simulink model "gm_sampleModel1847_5_sub"  (R2023a)
settings: Solver=VariableStepAuto  StartTime=0.0  StopTime=10.0  RelTol=1e-3
libraries: hdlsllib x1
settings Model: Creator=user1  LastModifiedBy=user1
settings OptimizationCC: BlockReduction=off  ConditionallyExecuteInputs=off
settings DebuggingCC: InheritedTsInSrcMsg=none

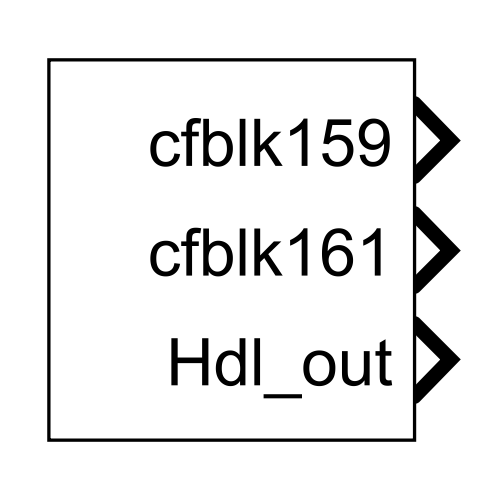
[thumbnail: Simulink's stored preview of the top-level diagram]
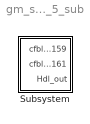
== system gm_sampleModel1847_5_sub ==
  Subsystem : Subsystem

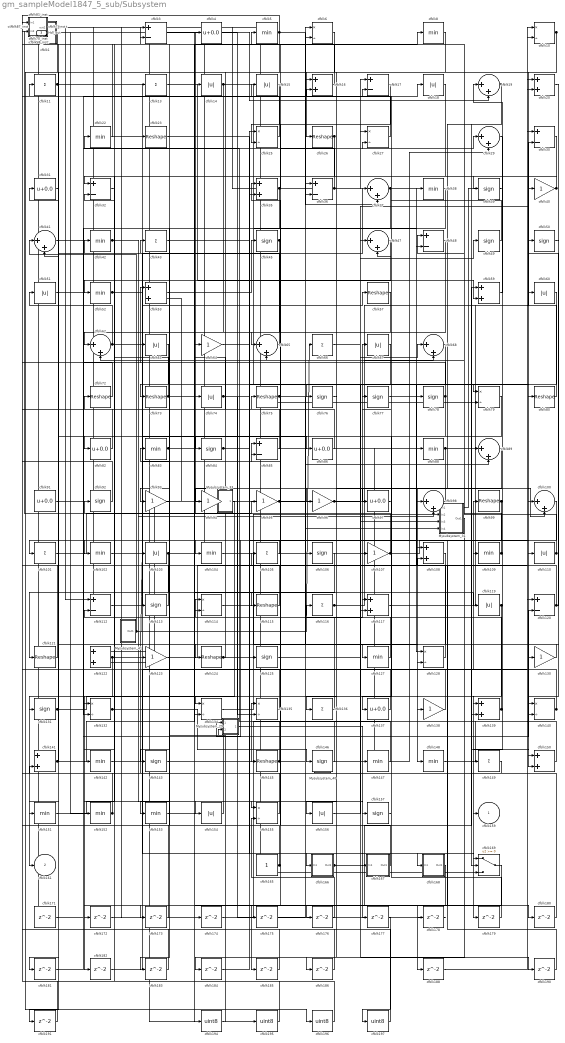
== system gm_sampleModel1847_5_sub/Subsystem ==
  Mysubsystem_29 : Subsystem
  Mysubsystem_31 : Subsystem
  Mysubsystem_33 : Subsystem
  Mysubsystem_40 : Subsystem
  Mysubsystem_41 : Subsystem
  cfblk1 : Subsystem  mask(Detect Fall Nonpositive){vinit=double(0), InputProcessing=Elements as channels (sample based), OutDataTypeStr=uint8}
      mask prompts: vinit "Simulink:masks:InitialCondition_MP"; InputProcessing "Simulink:masks:InputProcessing_MP"; OutDataTypeStr "Simulink:masks:OutputDataType_MP"
      mask help: Simulink:masks:DetectFallNonpositive_MD
      mask init:
      | InputProcessing = 'Elements as channels (sample based)';
      | OutDataTypeStr = 'uint8';
      | vinit = double(0);
      mask TypeOptions InputProcessing: Simulink:masks:ColumnsAsChannelsFrameBased | Simulink:masks:ElementsAsChannelsSampleBased
      mask TypeOptions OutDataTypeStr: Simulink:masks:uint8 | Simulink:masks:boolean
      mask Display: fprintf('U <= 0\n&  NOT\nU/z <= 0')
  cfblk{6,10,25,27,79,114,128,132,134..135,140,155} (12 alike) : Product  Inputs=*/  OutDataTypeStr=uint8  RndMeth=Zero  SaturateOnIntegerOverflow=on
  cfblk{19,29,37,41,47,62,65,68,89,98,100} (11 alike) : Sum  Inputs=|++  OutDataTypeStr=uint8
  cfblk{11,13,43,66,101,105,116,136,149} (9 alike) : Sum  Inputs=+  OutDataTypeStr=uint8
  cfblk{5,8,22,38,42,52,83,88,102,104,109,127,142,147..148,151..153} (18 alike) : MinMax  OutDataTypeStr=uint8
  cfblk{14..15,18,51,60,63,67,74,103,110,119,154,156} (13 alike) : Abs  OutDataTypeStr=uint8  SaturateOnIntegerOverflow=off
  cfblk{39,45,49..50,76..78,84,92,106,113,125,131,143,146,157} (16 alike) : Signum
  cfblk{40,64,93..96,107,123,130,138} (10 alike) : Gain  OutDataTypeStr=uint8
  cfblk{16,20,35,53,59,108,117,122,139,141,150} (11 alike) : Sum  OutDataTypeStr=uint8
  cfblk{3,17,30,32,36,48,85,112,120} (9 alike) : Sum  Inputs=+-  OutDataTypeStr=uint8
  cfblk{23,26,57,72..73,75,80,99,115,121,124,145} (12 alike) : Reshape
  cfblk12_inst : Subsystem
  cfblk133_inst : Subsystem
  cfblk{4,31,82,86,91,97,137} (7 alike) : Bias  Bias=0.0  SaturateOnIntegerOverflow=off
  cfblk144_inst : Subsystem
  cfblk165 : Constant  OutDataTypeStr=uint8  SampleTime=-1
  cfblk166 : Subsystem
  cfblk167 : Subsystem
  cfblk168 : Subsystem
  cfblk169 : Switch  OutDataTypeStr=uint8  SaturateOnIntegerOverflow=off  InputSameDT=off
  cfblk{171..186,188,190..191} (19 alike) : Delay  SampleTime=1
  cfblk{194..197} (4 alike) : DataTypeConversion  OutDataTypeStr=uint8  SaturateOnIntegerOverflow=off  RndMeth=Floor
  cfblk24_inst : Subsystem
  cfblk34_inst : Subsystem
  cfblk55_inst : Subsystem
  cfblk56_inst : Subsystem
  cfblk58_inst : Subsystem
  cfblk70_inst : Subsystem
  cfblk7_inst : Subsystem
  cfblk81_inst : Subsystem
  cfblk87_inst : Subsystem
  cfblk159 : Outport  OutDataTypeStr=uint8  SampleTime=1  VectorParamsAs1DForOutWhenUnconnected=off
  cfblk161 : Outport  Port=2  OutDataTypeStr=uint8  SampleTime=1  VectorParamsAs1DForOutWhenUnconnected=off
  Hdl_out : Outport  Port=3  OutDataTypeStr=uint8  SampleTime=1
  wires:
  Mysubsystem_29/1(Out1) -> cfblk177/1
  Mysubsystem_31/1(Out1) -> cfblk184/1
  Mysubsystem_33/1(cfblk161) -> cfblk161/1
  Mysubsystem_40/1(Out1) -> cfblk29/2, cfblk88/1
  Mysubsystem_41/1(Out1) -> cfblk41/1, cfblk66/1
  cfblk1/1(Y) -> cfblk196/1
  cfblk10/1 -> cfblk26/1, cfblk150/2
  cfblk100/1 -> cfblk104/1
  cfblk101/1 -> cfblk95/1
  cfblk102/1 -> cfblk85/1
  cfblk103/1 -> cfblk181/1, cfblk180/1
  cfblk104/1 -> cfblk127/1
  cfblk105/1 -> cfblk101/1
  cfblk106/1 -> cfblk121/1
  cfblk107/1 -> cfblk81_inst/2(in2), cfblk4/1, cfblk110/1
  cfblk108/1 -> cfblk151/1
  cfblk109/1 -> cfblk55_inst/2(in2), cfblk48/1
  cfblk11/1 -> cfblk86/1, cfblk16/2, cfblk157/1
  cfblk110/1 -> cfblk87_inst/2(in2), cfblk62/2
  cfblk112/1 -> cfblk57/1
  cfblk113/1 -> cfblk56_inst/1(in1)
  cfblk114/1 -> Mysubsystem_31/2(In2)
  cfblk115/1 -> cfblk105/1
  cfblk116/1 -> cfblk68/2, cfblk30/2
  cfblk117/1 -> cfblk60/1
  cfblk119/1 -> cfblk179/1, cfblk159/1
  cfblk12_inst/1(out1) -> cfblk13/1
  cfblk120/1 -> cfblk75/1, cfblk50/1
  cfblk121/1 -> cfblk87_inst/1(in1)
  cfblk122/1 -> cfblk103/1, cfblk182/1
  cfblk123/1 -> cfblk20/1
  cfblk124/1 -> cfblk78/1, cfblk74/1
  cfblk125/1 -> Mysubsystem_31/3(In3)
  cfblk127/1 -> cfblk116/1
  cfblk128/1 -> cfblk3/1
  cfblk13/1 -> cfblk59/2
  cfblk130/1 -> cfblk124/1
  cfblk131/1 -> cfblk139/1, cfblk134/1
  cfblk132/1 -> cfblk194/1, cfblk146/1
  cfblk133_inst/1(out1) -> cfblk174/1
  cfblk134/1 -> cfblk99/1
  cfblk135/1 -> cfblk51/1
  cfblk136/1 -> cfblk112/2
  cfblk137/1 -> cfblk144_inst/1(in1)
  cfblk138/1 -> cfblk92/1
  cfblk139/1 -> cfblk67/1, cfblk47/2
  cfblk14/1 -> cfblk48/2, cfblk132/1, cfblk147/1
  cfblk140/1 -> cfblk85/2, cfblk109/1
  cfblk141/1 -> cfblk31/1, cfblk8/1
  cfblk142/1 -> cfblk169/1
  cfblk143/1 -> cfblk135/1
  cfblk144_inst/1(out1) -> cfblk12_inst/2(in2), cfblk38/1
  cfblk145/1 -> cfblk89/2, cfblk72/1, cfblk65/2, cfblk117/1, Mysubsystem_31/4(In4)
  cfblk146/1 -> cfblk22/1
  cfblk147/1 -> cfblk114/1
  cfblk148/1 -> cfblk120/2
  cfblk149/1 -> cfblk141/2
  cfblk15/1 -> cfblk25/2
  cfblk150/1 -> cfblk30/1
  cfblk151/1 -> cfblk154/1
  cfblk152/1 -> cfblk133_inst/2(in2), Hdl_out/1
  cfblk153/1 -> cfblk168/1(In1)
  cfblk154/1 -> cfblk83/1
  cfblk155/1 -> cfblk123/1
  cfblk156/1 -> cfblk49/1
  cfblk157/1 -> cfblk77/1
  cfblk16/1 -> cfblk7_inst/2(in2)
  cfblk165/1 -> cfblk32/2, cfblk43/1
  cfblk166/1(Out1) -> cfblk139/2, cfblk188/1
  cfblk167/1(Out1) -> cfblk35/1
  cfblk168/1(Out1) -> cfblk172/1
  cfblk169/1 -> cfblk185/1
  cfblk17/1 -> cfblk65/1
  cfblk171/1 -> cfblk140/2
  cfblk172/1 -> cfblk36/1
  cfblk173/1 -> cfblk34_inst/1(in1)
  cfblk174/1 -> cfblk20/2
  cfblk175/1 -> cfblk6/2
  cfblk176/1 -> cfblk155/2
  cfblk177/1 -> cfblk197/1
  cfblk178/1 -> cfblk1/1(U)
  cfblk179/1 -> cfblk17/2
  cfblk18/1 -> cfblk76/1
  cfblk180/1 -> cfblk59/1
  cfblk181/1 -> cfblk27/2
  cfblk182/1 -> cfblk10/2
  cfblk183/1 -> cfblk81_inst/1(in1)
  cfblk184/1 -> cfblk35/2
  cfblk185/1 -> cfblk12_inst/1(in1)
  cfblk186/1 -> cfblk144_inst/2(in2)
  cfblk188/1 -> cfblk120/1
  cfblk19/1 -> cfblk169/2, cfblk148/1
  cfblk190/1 -> cfblk108/2
  cfblk191/1 -> cfblk56_inst/2(in2)
  cfblk194/1 -> Mysubsystem_29/2(In2)
  cfblk195/1 -> cfblk42/1
  cfblk196/1 -> cfblk58_inst/1(in1)
  cfblk197/1 -> cfblk58_inst/2(in2)
  cfblk20/1 -> cfblk140/1
  cfblk22/1 -> cfblk7_inst/1(in1)
  cfblk23/1 -> cfblk97/1
  cfblk24_inst/1(out1) -> cfblk89/1, cfblk112/1
  cfblk25/1 -> cfblk24_inst/2(in2)
  cfblk26/1 -> cfblk62/1, cfblk36/2
  cfblk27/1 -> cfblk6/1
  cfblk29/1 -> cfblk149/1
  cfblk3/1 -> cfblk166/1(In1)
  cfblk30/1 -> cfblk152/1
  cfblk31/1 -> cfblk131/1
  cfblk32/1 -> cfblk142/1
  cfblk34_inst/1(out1) -> cfblk113/1
  cfblk35/1 -> cfblk82/1, cfblk132/2, cfblk5/1
  cfblk36/1 -> cfblk17/1, cfblk15/1
  cfblk37/1 -> cfblk100/2, cfblk93/1
  cfblk38/1 -> cfblk153/1
  cfblk39/1 -> Mysubsystem_31/1(In1)
  cfblk4/1 -> cfblk19/2
  cfblk40/1 -> cfblk39/1, cfblk32/1
  cfblk41/1 -> cfblk29/1
  cfblk42/1 -> cfblk98/2, cfblk155/1
  cfblk43/1 -> cfblk145/1
  cfblk45/1 -> cfblk183/1, cfblk52/1
  cfblk47/1 -> cfblk134/2
  cfblk48/1 -> cfblk102/1
  cfblk49/1 -> cfblk14/1
  cfblk5/1 -> cfblk55_inst/1(in1), cfblk41/2, cfblk37/2
  cfblk50/1 -> cfblk130/1
  cfblk51/1 -> cfblk18/1
  cfblk52/1 -> cfblk106/1, cfblk114/2
  cfblk53/1 -> cfblk45/1
  cfblk55_inst/1(out1) -> cfblk23/1
  cfblk56_inst/1(out1) -> cfblk107/1
  cfblk57/1 -> cfblk175/1
  cfblk58_inst/1(out1) -> cfblk195/1
  cfblk59/1 -> cfblk19/1
  cfblk6/1 -> cfblk84/1
  cfblk60/1 -> cfblk94/1
  cfblk62/1 -> cfblk37/1, cfblk11/1
  cfblk63/1 -> cfblk73/1
  cfblk64/1 -> cfblk80/1
  cfblk65/1 -> cfblk34_inst/2(in2)
  cfblk66/1 -> cfblk47/1
  cfblk67/1 -> cfblk115/1
  cfblk68/1 -> cfblk143/1
  cfblk7_inst/1(out1) -> cfblk91/1
  cfblk70_inst/1(out1) -> cfblk125/1
  cfblk72/1 -> cfblk70_inst/1(in1)
  cfblk73/1 -> cfblk133_inst/1(in1), cfblk117/2
  cfblk74/1 -> cfblk108/1, cfblk135/2
  cfblk75/1 -> cfblk16/1, cfblk128/2
  cfblk76/1 -> cfblk136/1
  cfblk77/1 -> cfblk79/1
  cfblk78/1 -> cfblk53/1, cfblk191/1, cfblk128/1
  cfblk79/1 -> cfblk137/1
  cfblk8/1 -> cfblk176/1
  cfblk80/1 -> cfblk10/1
  cfblk81_inst/1(out1) -> cfblk79/2, cfblk171/1
  cfblk82/1 -> cfblk24_inst/1(in1)
  cfblk83/1 -> cfblk3/2, cfblk96/1, cfblk27/1
  cfblk84/1 -> cfblk138/1, cfblk167/1(In1)
  cfblk85/1 -> cfblk64/1
  cfblk86/1 -> cfblk25/1
  cfblk87_inst/1(out1) -> cfblk169/3, cfblk141/1
  cfblk88/1 -> cfblk156/1, cfblk150/1
  cfblk89/1 -> cfblk98/1
  cfblk91/1 -> cfblk63/1
  cfblk92/1 -> cfblk70_inst/2(in2)
  cfblk93/1 -> cfblk173/1
  cfblk94/1 -> cfblk53/2, cfblk122/2, cfblk122/1
  cfblk95/1 -> cfblk119/1, cfblk100/1
  cfblk96/1 -> cfblk68/1, cfblk40/1, cfblk190/1
  cfblk97/1 -> Mysubsystem_33/1(u)
  cfblk98/1 -> cfblk186/1
  cfblk99/1 -> cfblk178/1, Mysubsystem_29/1(In1)

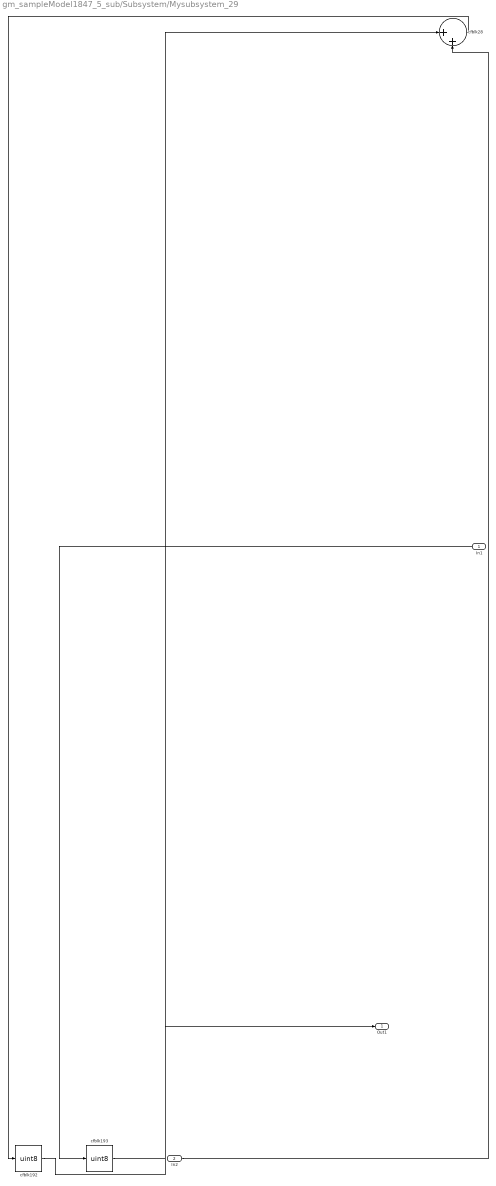
== system gm_sampleModel1847_5_sub/Subsystem/Mysubsystem_29 ==
  In1 : Inport  OutDataTypeStr=uint8  PortDimensions=1  SampleTime=1
  In2 : Inport  Port=2  OutDataTypeStr=uint8  PortDimensions=1  SampleTime=1
  cfblk192 : DataTypeConversion  OutDataTypeStr=uint8  SaturateOnIntegerOverflow=off  RndMeth=Floor
  cfblk193 : DataTypeConversion  OutDataTypeStr=uint8  SaturateOnIntegerOverflow=off  RndMeth=Floor
  cfblk28 : Sum  Inputs=|++
  Out1 : Outport  SampleTime=1
  wires:
  In1/1 -> cfblk193/1
  In2/1 -> cfblk28/2
  cfblk192/1 -> Out1/1
  cfblk193/1 -> cfblk28/1
  cfblk28/1 -> cfblk192/1

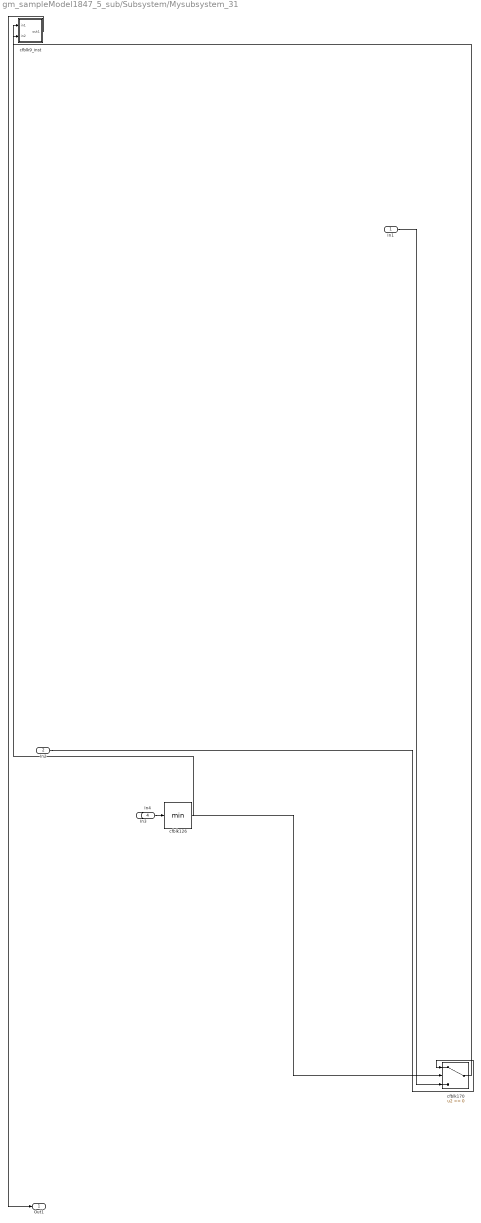
== system gm_sampleModel1847_5_sub/Subsystem/Mysubsystem_31 ==
  In1 : Inport  OutDataTypeStr=uint8  PortDimensions=1  SampleTime=1
  In2 : Inport  Port=2  OutDataTypeStr=uint8  PortDimensions=1  SampleTime=1
  In3 : Inport  Port=3  OutDataTypeStr=uint8  PortDimensions=1  SampleTime=1
  In4 : Inport  Port=4  OutDataTypeStr=uint8  PortDimensions=1  SampleTime=1
  cfblk126 : MinMax
  cfblk170 : Switch  SaturateOnIntegerOverflow=off  InputSameDT=off
  cfblk9_inst : Subsystem
  Out1 : Outport  SampleTime=1
  wires:
  In1/1 -> cfblk170/3
  In2/1 -> cfblk170/1
  In3/1 -> cfblk170/2
  In4/1 -> cfblk126/1
  cfblk126/1 -> cfblk9_inst/1(in1)
  cfblk170/1 -> cfblk9_inst/2(in2)
  cfblk9_inst/1(out1) -> Out1/1

== system gm_sampleModel1847_5_sub/Subsystem/Mysubsystem_33 ==
  u : Inport  OutDataTypeStr=uint8  PortDimensions=1  SampleTime=1
  cfblk2 : hdlsllib/Logic and Bit Operations/Bit Slice  lidx=7  ridx=0
  cfblk161 : Outport  SampleTime=1  VectorParamsAs1DForOutWhenUnconnected=off
  wires:
  u/1 -> cfblk2/1
  cfblk2/1 -> cfblk161/1

== system gm_sampleModel1847_5_sub/Subsystem/Mysubsystem_40 ==
  cfblk129 : Abs  SaturateOnIntegerOverflow=off
  cfblk163 : Subsystem  mask(Counter Limited){uplimit=double(7), tsamp=double(-1)}
      mask prompts: uplimit "Simulink:masks:UpperLimit_MP"; tsamp "Simulink:masks:SampleTime_MP"
      mask help: Simulink:masks:CounterLimited_MD
      mask init:
      | nbits = double(8);
      | tsamp = double(-1);
      | uplimit = double(7);
  Out1 : Outport  SampleTime=1
  wires:
  cfblk129/1 -> Out1/1
  cfblk163/1(y) -> cfblk129/1

== system gm_sampleModel1847_5_sub/Subsystem/Mysubsystem_41 ==
  cfblk164 : Ground
  cfblk71 : Signum
  Out1 : Outport  SampleTime=1
  wires:
  cfblk164/1 -> cfblk71/1
  cfblk71/1 -> Out1/1

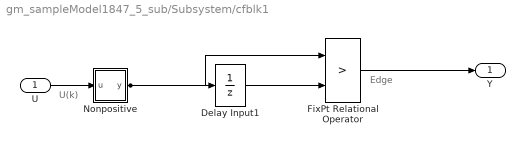
== system gm_sampleModel1847_5_sub/Subsystem/cfblk1 ==
  note: U(k)
  note: Edge
  U : Inport  OutDataTypeStr=uint8  SampleTime=1
  Delay Input1 : UnitDelay  Description=Store in Global RAM  DisableCoverage=on  InitialCondition=vinit  SampleTime=-1  HasFrameUpgradeWarning=on
  FixPt Relational Operator : RelationalOperator  Operator=>  OutDataTypeStr=fixdt(0, 8)  ZeroCross=off  InputSameDT=off
  Nonpositive : Subsystem  mask(Compare To Zero){relop=<=, OutDataTypeStr=boolean, ZeroCross=off}
      mask prompts: relop "Simulink:masks:Operator_MP"; OutDataTypeStr "Simulink:masks:OutputDataType_MP"; ZeroCross "Simulink:masks:EnableZerocrossingDetection_MP"
      mask help: Simulink:masks:CompareToZero_MD
      mask init:
      | OutDataTypeStr = 'boolean';
      | ZeroCross = 'off';
      | blkName = 'sampleModel1847_5_sub/Subsystem/cfblk1/Nonpositive';
      | relop = '<=';
      | setValue = 'boolean';
      mask TypeOptions relop: == | ~= | < | <= | >= | >
      mask TypeOptions OutDataTypeStr: Simulink:masks:uint8 | Simulink:masks:boolean
      mask Callback ZeroCross: sl('zeroCrossEnable', gcbh);
      mask Display: disp([relop,' 0'])
  Y : Outport  SampleTime=1
  wires:
  U/1 -> Nonpositive/1(u)
  Delay Input1/1 -> FixPt Relational Operator/2
  FixPt Relational Operator/1 -> Y/1
  Nonpositive/1(y) -> FixPt Relational Operator/1, Delay Input1/1

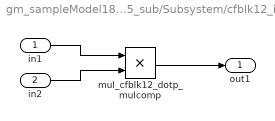
== system gm_sampleModel1847_5_sub/Subsystem/cfblk12_inst ==
  in1 : Inport  OutDataTypeStr=uint8  SampleTime=1
  in2 : Inport  Port=2  OutDataTypeStr=uint8  SampleTime=1
  mul_cfblk12_dotp_mulcomp : Product  Inputs=**  OutDataTypeStr=uint8  SampleTime=1
  out1 : Outport  OutDataTypeStr=uint8  SampleTime=1
  wires:
  in1/1 -> mul_cfblk12_dotp_mulcomp/1
  in2/1 -> mul_cfblk12_dotp_mulcomp/2
  mul_cfblk12_dotp_mulcomp/1 -> out1/1

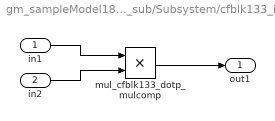
== system gm_sampleModel1847_5_sub/Subsystem/cfblk133_inst ==
  in1 : Inport  OutDataTypeStr=uint8  SampleTime=1
  in2 : Inport  Port=2  OutDataTypeStr=uint8  SampleTime=1
  mul_cfblk133_dotp_mulcomp : Product  Inputs=**  OutDataTypeStr=uint8  SampleTime=1
  out1 : Outport  OutDataTypeStr=uint8  SampleTime=1
  wires:
  in1/1 -> mul_cfblk133_dotp_mulcomp/1
  in2/1 -> mul_cfblk133_dotp_mulcomp/2
  mul_cfblk133_dotp_mulcomp/1 -> out1/1

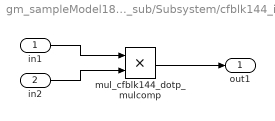
== system gm_sampleModel1847_5_sub/Subsystem/cfblk144_inst ==
  in1 : Inport  OutDataTypeStr=uint8  SampleTime=1
  in2 : Inport  Port=2  OutDataTypeStr=uint8  SampleTime=1
  mul_cfblk144_dotp_mulcomp : Product  Inputs=**  OutDataTypeStr=uint8  SampleTime=1
  out1 : Outport  OutDataTypeStr=uint8  SampleTime=1
  wires:
  in1/1 -> mul_cfblk144_dotp_mulcomp/1
  in2/1 -> mul_cfblk144_dotp_mulcomp/2
  mul_cfblk144_dotp_mulcomp/1 -> out1/1

== system gm_sampleModel1847_5_sub/Subsystem/cfblk166 ==
  In1 : Inport  OutDataTypeStr=uint8  PortDimensions=1  SampleTime=1
  Out1 : Outport  SampleTime=1
  wires:
  In1/1 -> Out1/1

== system gm_sampleModel1847_5_sub/Subsystem/cfblk167 ==
  In1 : Inport  OutDataTypeStr=uint8  PortDimensions=1  SampleTime=1
  Out1 : Outport  SampleTime=1
  wires:
  In1/1 -> Out1/1

== system gm_sampleModel1847_5_sub/Subsystem/cfblk168 ==
  In1 : Inport  OutDataTypeStr=uint8  PortDimensions=1  SampleTime=1
  Out1 : Outport  SampleTime=1
  wires:
  In1/1 -> Out1/1

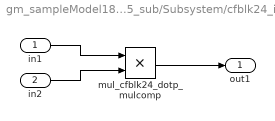
== system gm_sampleModel1847_5_sub/Subsystem/cfblk24_inst ==
  in1 : Inport  OutDataTypeStr=uint8  SampleTime=1
  in2 : Inport  Port=2  OutDataTypeStr=uint8  SampleTime=1
  mul_cfblk24_dotp_mulcomp : Product  Inputs=**  OutDataTypeStr=uint8  SampleTime=1
  out1 : Outport  OutDataTypeStr=uint8  SampleTime=1
  wires:
  in1/1 -> mul_cfblk24_dotp_mulcomp/1
  in2/1 -> mul_cfblk24_dotp_mulcomp/2
  mul_cfblk24_dotp_mulcomp/1 -> out1/1

== system gm_sampleModel1847_5_sub/Subsystem/cfblk34_inst ==
  in1 : Inport  OutDataTypeStr=uint8  SampleTime=1
  in2 : Inport  Port=2  OutDataTypeStr=uint8  SampleTime=1
  mul_cfblk34_dotp_mulcomp : Product  Inputs=**  OutDataTypeStr=uint8  SampleTime=1
  out1 : Outport  OutDataTypeStr=uint8  SampleTime=1
  wires:
  in1/1 -> mul_cfblk34_dotp_mulcomp/1
  in2/1 -> mul_cfblk34_dotp_mulcomp/2
  mul_cfblk34_dotp_mulcomp/1 -> out1/1

== system gm_sampleModel1847_5_sub/Subsystem/cfblk55_inst ==
  in1 : Inport  OutDataTypeStr=uint8  SampleTime=1
  in2 : Inport  Port=2  OutDataTypeStr=uint8  SampleTime=1
  mul_cfblk55_dotp_mulcomp : Product  Inputs=**  OutDataTypeStr=uint8  SampleTime=1
  out1 : Outport  OutDataTypeStr=uint8  SampleTime=1
  wires:
  in1/1 -> mul_cfblk55_dotp_mulcomp/1
  in2/1 -> mul_cfblk55_dotp_mulcomp/2
  mul_cfblk55_dotp_mulcomp/1 -> out1/1

== system gm_sampleModel1847_5_sub/Subsystem/cfblk56_inst ==
  in1 : Inport  OutDataTypeStr=uint8  SampleTime=1
  in2 : Inport  Port=2  OutDataTypeStr=uint8  SampleTime=1
  mul_cfblk56_dotp_mulcomp : Product  Inputs=**  OutDataTypeStr=uint8  SampleTime=1
  out1 : Outport  OutDataTypeStr=uint8  SampleTime=1
  wires:
  in1/1 -> mul_cfblk56_dotp_mulcomp/1
  in2/1 -> mul_cfblk56_dotp_mulcomp/2
  mul_cfblk56_dotp_mulcomp/1 -> out1/1

== system gm_sampleModel1847_5_sub/Subsystem/cfblk58_inst ==
  in1 : Inport  OutDataTypeStr=uint8  SampleTime=1
  in2 : Inport  Port=2  OutDataTypeStr=uint8  SampleTime=1
  mul_cfblk58_dotp_mulcomp : Product  Inputs=**  OutDataTypeStr=uint8  SampleTime=1
  out1 : Outport  OutDataTypeStr=uint8  SampleTime=1
  wires:
  in1/1 -> mul_cfblk58_dotp_mulcomp/1
  in2/1 -> mul_cfblk58_dotp_mulcomp/2
  mul_cfblk58_dotp_mulcomp/1 -> out1/1

== system gm_sampleModel1847_5_sub/Subsystem/cfblk70_inst ==
  in1 : Inport  OutDataTypeStr=uint8  SampleTime=1
  in2 : Inport  Port=2  OutDataTypeStr=uint8  SampleTime=1
  mul_cfblk70_dotp_mulcomp : Product  Inputs=**  OutDataTypeStr=uint8  SampleTime=1
  out1 : Outport  OutDataTypeStr=uint8  SampleTime=1
  wires:
  in1/1 -> mul_cfblk70_dotp_mulcomp/1
  in2/1 -> mul_cfblk70_dotp_mulcomp/2
  mul_cfblk70_dotp_mulcomp/1 -> out1/1

== system gm_sampleModel1847_5_sub/Subsystem/cfblk7_inst ==
  in1 : Inport  OutDataTypeStr=uint8  SampleTime=1
  in2 : Inport  Port=2  OutDataTypeStr=uint8  SampleTime=1
  mul_cfblk7_dotp_mulcomp : Product  Inputs=**  OutDataTypeStr=uint8  SampleTime=1
  out1 : Outport  OutDataTypeStr=uint8  SampleTime=1
  wires:
  in1/1 -> mul_cfblk7_dotp_mulcomp/1
  in2/1 -> mul_cfblk7_dotp_mulcomp/2
  mul_cfblk7_dotp_mulcomp/1 -> out1/1

== system gm_sampleModel1847_5_sub/Subsystem/cfblk81_inst ==
  in1 : Inport  OutDataTypeStr=uint8  SampleTime=1
  in2 : Inport  Port=2  OutDataTypeStr=uint8  SampleTime=1
  mul_cfblk81_dotp_mulcomp : Product  Inputs=**  OutDataTypeStr=uint8  SampleTime=1
  out1 : Outport  OutDataTypeStr=uint8  SampleTime=1
  wires:
  in1/1 -> mul_cfblk81_dotp_mulcomp/1
  in2/1 -> mul_cfblk81_dotp_mulcomp/2
  mul_cfblk81_dotp_mulcomp/1 -> out1/1

== system gm_sampleModel1847_5_sub/Subsystem/cfblk87_inst ==
  in1 : Inport  OutDataTypeStr=uint8  SampleTime=1
  in2 : Inport  Port=2  OutDataTypeStr=uint8  SampleTime=1
  mul_cfblk87_dotp_mulcomp : Product  Inputs=**  OutDataTypeStr=uint8  SampleTime=1
  out1 : Outport  OutDataTypeStr=uint8  SampleTime=1
  wires:
  in1/1 -> mul_cfblk87_dotp_mulcomp/1
  in2/1 -> mul_cfblk87_dotp_mulcomp/2
  mul_cfblk87_dotp_mulcomp/1 -> out1/1

== system gm_sampleModel1847_5_sub/Subsystem/Mysubsystem_31/cfblk9_inst ==
  in1 : Inport  OutDataTypeStr=uint8  SampleTime=1
  in2 : Inport  Port=2  OutDataTypeStr=uint8  SampleTime=1
  mul_cfblk9_dotp_mulcomp : Product  Inputs=**  OutDataTypeStr=uint16  SampleTime=1
  out1 : Outport  OutDataTypeStr=uint16  SampleTime=1
  wires:
  in1/1 -> mul_cfblk9_dotp_mulcomp/1
  in2/1 -> mul_cfblk9_dotp_mulcomp/2
  mul_cfblk9_dotp_mulcomp/1 -> out1/1

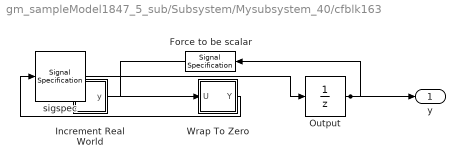
== system gm_sampleModel1847_5_sub/Subsystem/Mysubsystem_40/cfblk163 ==
  Force to be scalar : SignalSpecification  DisableCoverage=on  Dimensions=1
  Increment Real World : Subsystem  mask(Real World Value Increment){}
      mask help: Simulink:masks:RealWorldValueIncrement_MD
      mask Display: disp('V++')
  Output : UnitDelay  InitialCondition=0.0  SampleTime=tsamp  HasFrameUpgradeWarning=on
  Wrap To Zero : Subsystem  mask(Wrap To Zero){Threshold=double(7)}
      mask prompts: Threshold "Simulink:masks:Threshold_MP"
      mask help: Simulink:masks:WrapToZero_MD
  sigspec : SignalSpecification  OutDataTypeStr=uint8  Dimensions=1
  y : Outport  SampleTime=1
  wires:
  Force to be scalar/1 -> Increment Real World/1(u)
  Increment Real World/1(y) -> Wrap To Zero/1(U)
  Output/1 -> Force to be scalar/1, y/1
  Wrap To Zero/1(Y) -> sigspec/1
  sigspec/1 -> Output/1

== system gm_sampleModel1847_5_sub/Subsystem/cfblk1/Nonpositive ==
  u : Inport  OutDataTypeStr=uint8  SampleTime=1
  Compare : RelationalOperator  Operator=<=  OutDataTypeStr=boolean  ZeroCross=off
  Constant : Constant  DisableCoverage=on  Value=0  OutDataTypeStr=Inherit: Inherit via back propagation  SampleTime=-1  PreserveConstantTs=on
  y : Outport  SampleTime=1
  wires:
  u/1 -> Compare/1
  Compare/1 -> y/1
  Constant/1 -> Compare/2

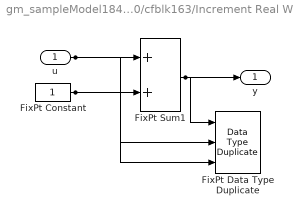
== system gm_sampleModel1847_5_sub/Subsystem/Mysubsystem_40/cfblk163/Increment Real World ==
  u : Inport  OutDataTypeStr=uint8  SampleTime=1
  FixPt Constant : Constant  DisableCoverage=on  OutDataTypeStr=Inherit: Inherit via back propagation  SampleTime=-1
  FixPt Data Type Duplicate : DataTypeDuplicate  DisableCoverage=on  NumInputPorts=3
  FixPt Sum1 : Sum  InputSameDT=on  OutDataTypeStr=Inherit: Inherit via back propagation  LockScale=on
  y : Outport  SampleTime=1
  wires:
  u/1 -> FixPt Sum1/1, FixPt Data Type Duplicate/2
  FixPt Constant/1 -> FixPt Sum1/2, FixPt Data Type Duplicate/3
  FixPt Sum1/1 -> FixPt Data Type Duplicate/1, y/1

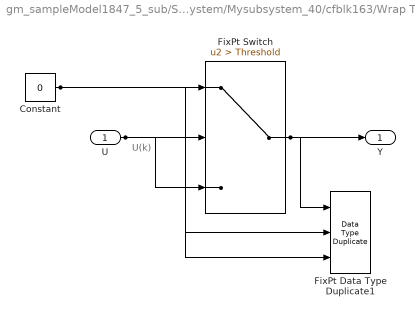
== system gm_sampleModel1847_5_sub/Subsystem/Mysubsystem_40/cfblk163/Wrap To Zero ==
  note: U(k)
  U : Inport  OutDataTypeStr=uint8  SampleTime=1
  Constant : Constant  DisableCoverage=on  Value=0  OutDataTypeStr=Inherit: Inherit via back propagation  SampleTime=-1
  FixPt Data Type Duplicate1 : DataTypeDuplicate  DisableCoverage=on  NumInputPorts=3
  FixPt Switch : Switch  Criteria=u2 > Threshold  Threshold=Threshold  OutDataTypeStr=Inherit: Inherit via back propagation  ZeroCross=off  SaturateOnIntegerOverflow=off  InputSameDT=off
  Y : Outport  SampleTime=1
  wires:
  U/1 -> FixPt Switch/3, FixPt Switch/2, FixPt Data Type Duplicate1/2
  Constant/1 -> FixPt Switch/1, FixPt Data Type Duplicate1/3
  FixPt Switch/1 -> FixPt Data Type Duplicate1/1, Y/1
